simulink model "project_part3_simulation_kalman"  (R2024a)
settings: Solver=VariableStepAuto  StartTime=0.0  StopTime=10.0  RelTol=1e-3
undefined symbols (not defined in the file): b, Continuous, J, K, Kc, L, Nbar, R, Time
libraries: simulink x2, ctrlSharedLib x1
settings Model: Creator=Harish  LastModifiedBy=Harish

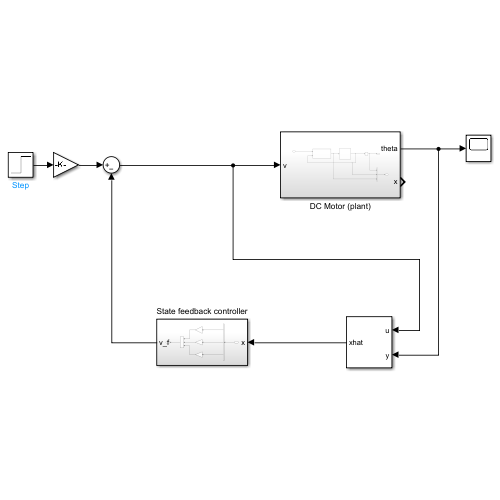
[thumbnail: Simulink's stored preview of the top-level diagram]
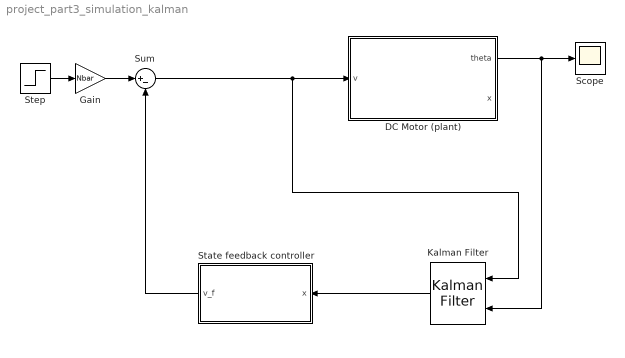
== system project_part3_simulation_kalman ==
  DC Motor (plant) : Subsystem
  Gain : Gain  Gain=Nbar
  Kalman Filter : ctrlSharedLib/Kalman Filter  TimeDomain=Continuous-Time  UseCurrentEstimator=on  ModelSource=LTI State-Space Variable  ModelSourceVariable=dcMotorSS  A=0.95  B=1  C=1  D=0  NumberOfStates=1  NumberOfInputs=1  NumberOfOutputs=1  InitialEstimateSource=Dialog  X0=0  P0=10  UseK=off  UseGH=off  NumberOfProcessNoiseInputs=1  G=1  TimeInvariantG=on  H=0  TimeInvariantH=on  Q=10  TimeInvariantQ=on  R=1  TimeInvariantR=on  N=0  TimeInvariantN=on  AddInputPort=on  AddEnablePort=off  OutputEstimatedY=off  OutputP=off  Ts=-1
  Scope : Scope
  State feedback controller : Subsystem
  Step : Step  SampleTime=0
  Sum : Sum  Inputs=|+-
  wires:
  DC Motor (plant)/1(theta) -> Kalman Filter/2, Scope/1
  Kalman Filter/1 -> State feedback controller/1(x)
  Step/1 -> Gain/1
  State feedback controller/1(v_f) -> Sum/2
  Sum/1 -> Kalman Filter/1, DC Motor (plant)/1(v)
  Gain/1 -> Sum/1

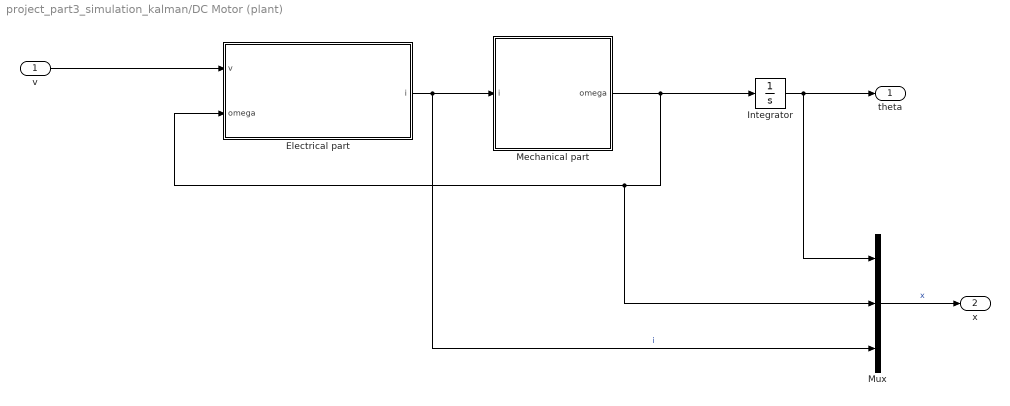
== system project_part3_simulation_kalman/DC Motor (plant) ==
  v : Inport
  "Electrical part " : Subsystem
  Integrator : Integrator
  Mechanical part : Subsystem
  Mux : Mux  Inputs=3
  theta : Outport
  x : Outport  Port=2
  wires:
  "Electrical part "/1(i) -> Mux/3, Mechanical part/1(i)  "i"
  Mechanical part/1(omega) -> Integrator/1, Mux/2, "Electrical part "/2(omega)
  v/1 -> "Electrical part "/1(v)
  Mux/1 -> x/1  "x"
  Integrator/1 -> Mux/1, theta/1

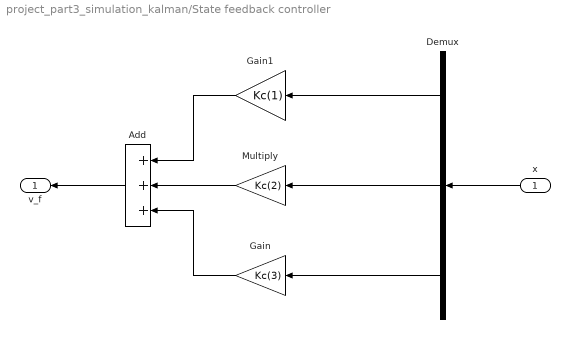
== system project_part3_simulation_kalman/State feedback controller ==
  x : Inport
  Add : Sum  Inputs=+++
  Demux : Demux  Outputs=3
  Gain : Gain  Gain=Kc(3)
  Gain1 : Gain  Gain=Kc(1)
  Multiply : Gain  Gain=Kc(2)
  v_f : Outport
  wires:
  Add/1 -> v_f/1
  x/1 -> Demux/1
  Demux/1 -> Gain1/1
  Demux/2 -> Multiply/1
  Demux/3 -> Gain/1
  Multiply/1 -> Add/2
  Gain1/1 -> Add/1
  Gain/1 -> Add/3

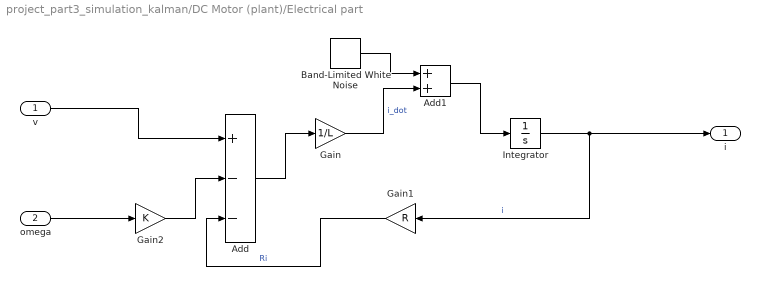
== system project_part3_simulation_kalman/DC Motor (plant)/Electrical part  ==
  v : Inport
  omega : Inport  Port=2
  Add : Sum  Inputs=+--
  Add1 : Sum
  Band-Limited White Noise : simulink/Sources/Band-Limited White Noise  Cov=10*0.001  Ts=0.001  seed=25
  Gain : Gain  Gain=1/L
  Gain1 : Gain  Gain=R
  Gain2 : Gain  Gain=K
  Integrator : Integrator  InitialCondition=0.5
  i : Outport
  wires:
  Add/1 -> Gain/1
  Integrator/1 -> i/1, Gain1/1  "i"
  Gain1/1 -> Add/3  "Ri"
  v/1 -> Add/1
  Gain2/1 -> Add/2
  omega/1 -> Gain2/1
  Band-Limited White Noise/1 -> Add1/1
  Gain/1 -> Add1/2  "i_dot"
  Add1/1 -> Integrator/1

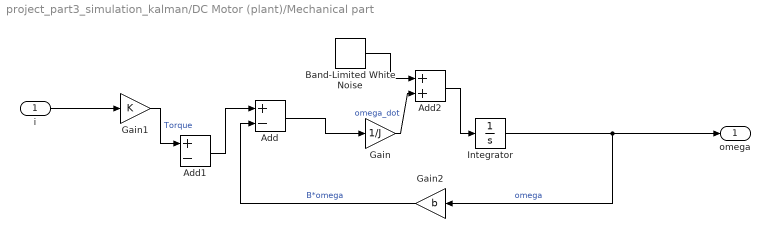
== system project_part3_simulation_kalman/DC Motor (plant)/Mechanical part ==
  i : Inport
  Add : Sum  Inputs=+-
  Add1 : Sum  Inputs=+-
  Add2 : Sum
  Band-Limited White Noise : simulink/Sources/Band-Limited White Noise  Cov=10*0.001  Ts=0.001  seed=25
  Gain : Gain  Gain=1/J
  Gain1 : Gain  Gain=K
  Gain2 : Gain  Gain=b
  Integrator : Integrator  InitialCondition=0.05
  omega : Outport
  wires:
  Add/1 -> Gain/1
  Integrator/1 -> omega/1, Gain2/1  "omega"
  Gain2/1 -> Add/2  "B*omega"
  i/1 -> Gain1/1
  Gain1/1 -> Add1/1  "Torque"
  Add1/1 -> Add/1
  Band-Limited White Noise/1 -> Add2/1
  Gain/1 -> Add2/2  "omega_dot"
  Add2/1 -> Integrator/1
